simulink model "pid_controller_project"  (R2024b)
settings: Solver=VariableStepAuto  StartTime=0.0  StopTime=70  RelTol=1e-3
values from neighbouring files (symbols this model uses):
  A = pi*1    (= 3.14159265359)    [project_pid_controller.m]
  c = 0.6*sqrt(2*9.81)    [project_pid_controller.m]
  Kd = 0.0001    [project_pid_controller.m]
  Kd_filter = 0.05*Kd    (= 5e-06)    [project_pid_controller.m]
  Ki = 0.2    [project_pid_controller.m]
  Kp = 0.5    [project_pid_controller.m]
settings Model: Creator=lenovo  LastModifiedBy=lenovo

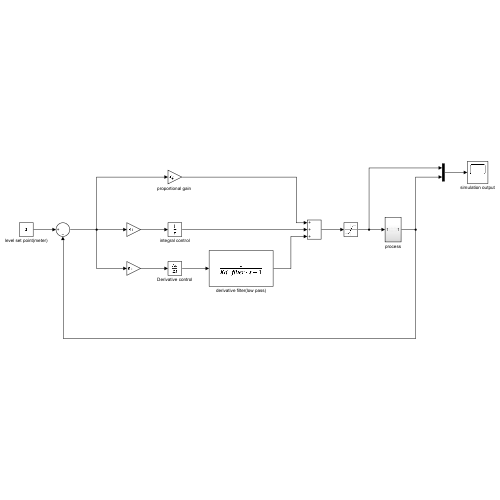
[thumbnail: Simulink's stored preview of the top-level diagram]
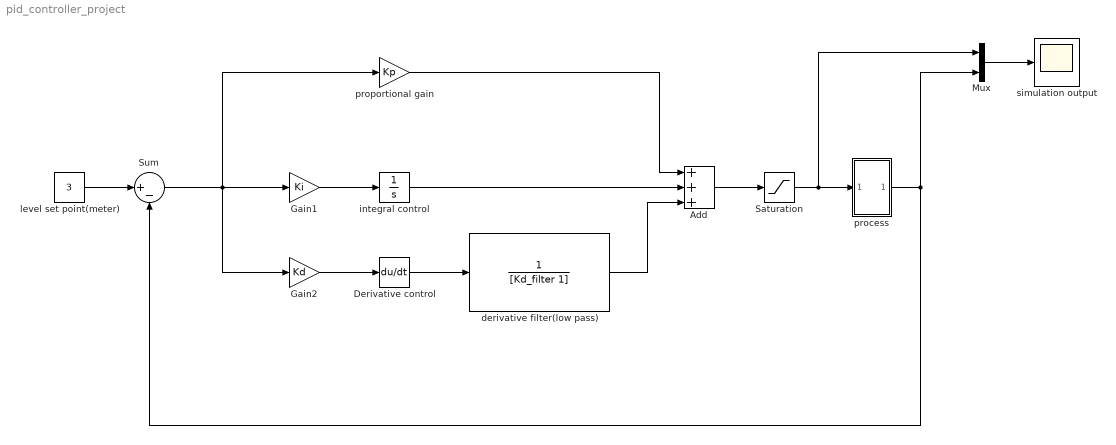
== system pid_controller_project ==
  Add : Sum  Inputs=+++
  Derivative control : Derivative
  Gain1 : Gain  Gain=Ki
  Gain2 : Gain  Gain=Kd
  Mux : Mux  Inputs=2
  Saturation : Saturate  UpperLimit=10  LowerLimit=0
  Sum : Sum  Inputs=|+-
  derivative filter(low pass) : TransferFcn  Denominator=[Kd_filter 1]
  integral control : Integrator
  level set point(meter) : Constant  Value=3
  process : Subsystem
  "proportional gain " : Gain  Gain=Kp
  simulation output : Scope
  wires:
  process/1(Out1) -> Sum/2, Mux/2
  level set point(meter)/1 -> Sum/1
  Saturation/1 -> process/1(In1), Mux/1
  Add/1 -> Saturation/1
  Sum/1 -> Gain2/1, Gain1/1, "proportional gain "/1
  "proportional gain "/1 -> Add/1
  Gain1/1 -> integral control/1
  integral control/1 -> Add/2
  Gain2/1 -> Derivative control/1
  Derivative control/1 -> derivative filter(low pass)/1
  derivative filter(low pass)/1 -> Add/3
  Mux/1 -> simulation output/1

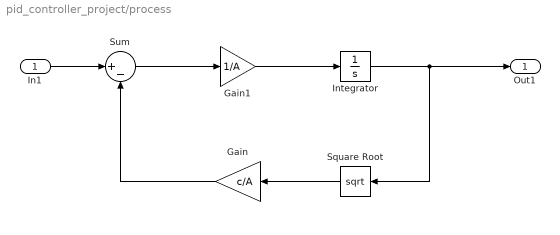
== system pid_controller_project/process ==
  In1 : Inport
  Gain : Gain  Gain=c/A
  Gain1 : Gain  Gain=1/A
  Integrator : Integrator
  Square Root : Sqrt
  Sum : Sum  Inputs=|+-
  Out1 : Outport
  wires:
  Square Root/1 -> Gain/1
  Gain1/1 -> Integrator/1
  Sum/1 -> Gain1/1
  In1/1 -> Sum/1
  Integrator/1 -> Out1/1, Square Root/1
  Gain/1 -> Sum/2
